simulink library "findTargetPathParameter"  (R2022a)
settings: Solver=VariableStepAuto  StartTime=0.0  StopTime=10.0  RelTol=1e-3
undefined symbols (not defined in the file or in its folder): convergeTol
libraries: calcDistanceFromPath x4, calcPathLengthOverRange x3
settings Model: Creator=Ayaz  LastModifiedBy=lhill8
settings SolverCC: AlgebraicLoopSolver=TrustRegion
settings DebuggingCC: UnconnectedInputMsg=warning  UnconnectedOutputMsg=warning  UnconnectedLineMsg=warning  SFMachineParentedDataDiag=warning

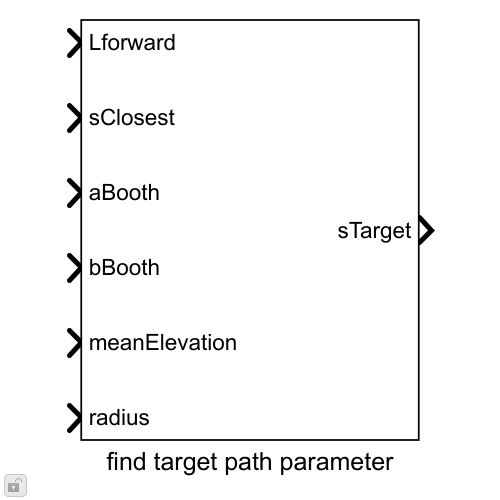
[thumbnail: Simulink's stored preview of the top-level diagram]
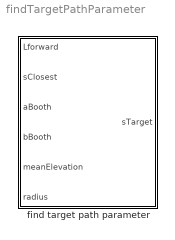
== system findTargetPathParameter ==
  find target path parameter : Subsystem  mask{maxBackward=0, maxForward=0.25, tau=0.618, convergeTol=convergeTol, MaxIters=25}
      mask prompts: maxBackward "Maximum normalized backward search"; maxForward "Maximum normalized forward search"; tau "Golden ratio"; convergeTol "Convergence tolerance"; MaxIters "Maximum number of iterations"
      mask TypeOptions maxBackward: Constant/Value
      mask TypeOptions maxForward: Constant1/Value
      mask TypeOptions tau: Golden section search/tau
      mask TypeOptions convergeTol: Golden section search/convergeTol
      mask TypeOptions MaxIters: Golden section search/MaxIters

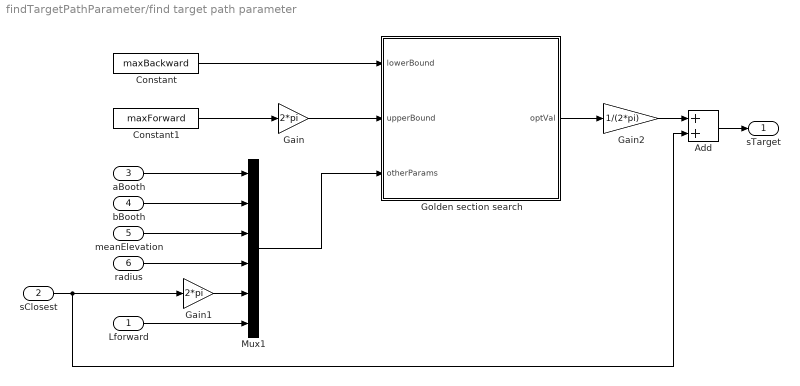
== system findTargetPathParameter/find target path parameter ==
  Lforward : Inport
  sClosest : Inport  Port=2
  aBooth : Inport  Port=3
  bBooth : Inport  Port=4
  meanElevation : Inport  Port=5
  radius : Inport  Port=6
  Add : Sum
  Constant : Constant  Value=maxBackward
  Constant1 : Constant  Value=maxForward
  Gain : Gain  Gain=2*pi
  Gain1 : Gain  Gain=2*pi
  Gain2 : Gain  Gain=1/(2*pi)
  Golden section search : Subsystem  TreatAsAtomicUnit=on  mask{tau=tau, convergeTol=convergeTol, MaxIters=25}
      mask prompts: tau "Golden ratio"; convergeTol "Convergence tolerance"; MaxIters "Maximum number of iterations"
      mask TypeOptions tau: GS initialization/tau | GS update/tau
      mask TypeOptions convergeTol: Constant/Value
      mask TypeOptions MaxIters: While Iterator/MaxIters
  Mux1 : Mux  Inputs=6
  sTarget : Outport
  wires:
  Golden section search/1(optVal) -> Gain2/1
  aBooth/1 -> Mux1/1
  radius/1 -> Mux1/4
  sClosest/1 -> Add/2, Gain1/1
  meanElevation/1 -> Mux1/3
  bBooth/1 -> Mux1/2
  Lforward/1 -> Mux1/6
  Mux1/1 -> Golden section search/3(otherParams)
  Constant/1 -> Golden section search/1(lowerBound)
  Constant1/1 -> Gain/1
  Gain/1 -> Golden section search/2(upperBound)
  Gain1/1 -> Mux1/5
  Gain2/1 -> Add/1
  Add/1 -> sTarget/1

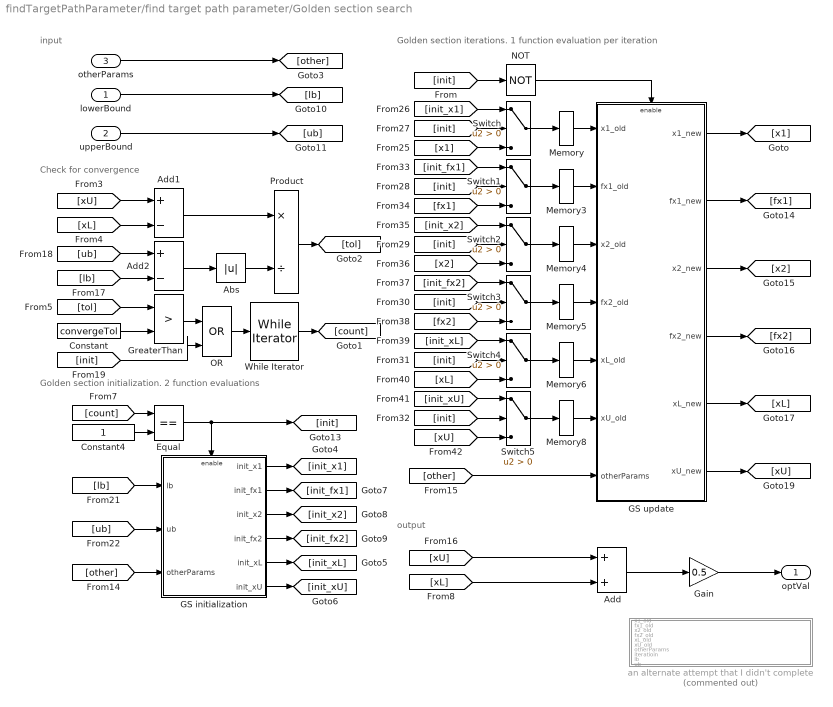
== system findTargetPathParameter/find target path parameter/Golden section search ==
  note: input
  note: output
  note: Golden section iterations. 1 function evaluation per iteration
  note: Golden section initialization. 2 function evaluations
  note: Check for convergence
  lowerBound : Inport
  upperBound : Inport  Port=2
  otherParams : Inport  Port=3
  Abs : Abs  SaturateOnIntegerOverflow=off
  Add : Sum
  Add1 : Sum  Inputs=+-
  Add2 : Sum  Inputs=+-
  Constant : Constant  Value=convergeTol
  Constant4 : Constant
  Equal : RelationalOperator  Operator===  OutDataTypeStr=boolean  RndMeth=Simplest  InputSameDT=off
  GS initialization : Subsystem  TreatAsAtomicUnit=on  mask{tau=tau}
      mask prompts: tau "Golden ratio"
      mask TypeOptions tau: Gain/Gain
  GS update : Subsystem  TreatAsAtomicUnit=on  mask{tau=tau}
      mask prompts: tau "Golden ratio"
      mask TypeOptions tau: Gain/Gain | Gain1/Gain
  Gain : Gain  Gain=0.5
  GreaterThan : RelationalOperator  Operator=>  OutDataTypeStr=boolean  RndMeth=Simplest  InputSameDT=off
  Memory{,3..6,8} (6 alike) : Memory  InheritSampleTime=on
  NOT : Logic  Operator=NOT  IconShape=distinctive  AllPortsSameDT=off  OutDataTypeStr=boolean
  OR : Logic  Operator=OR  IconShape=distinctive  AllPortsSameDT=off  OutDataTypeStr=boolean
  Product : Product  Inputs=*/
  Switch{,1..5} (6 alike) : Switch  Criteria=u2 > Threshold  SaturateOnIntegerOverflow=off  InputSameDT=off
  While Iterator : WhileIterator  MaxIters=MaxIters  WhileBlockType=do-while  ResetStates=reset  ShowIterationPort=on
  an alternate attempt that I didn't complete : Subsystem  Commented=on
  optVal : Outport
  wires:
  GreaterThan/1 -> OR/1
  Gain/1 -> optVal/1
  While Iterator/1 -> [count]
  [count] -> Equal/1
  Constant4/1 -> Equal/2
  Equal/1 -> [init], GS initialization/Enable
  [init] -> NOT/1
  Add/1 -> Gain/1
  GS initialization/1(init_x1) -> [init_x1]
  GS initialization/2(init_fx1) -> [init_fx1]
  GS initialization/3(init_x2) -> [init_x2]
  GS initialization/4(init_fx2) -> [init_fx2]
  GS update/1(x1_new) -> [x1]
  GS update/2(fx1_new) -> [fx1]
  GS update/3(x2_new) -> [x2]
  GS update/5(xL_new) -> [xL]
  GS update/6(xU_new) -> [xU]
  GS update/4(fx2_new) -> [fx2]
  otherParams/1 -> [other]
  GS initialization/5(init_xL) -> [init_xL]
  GS initialization/6(init_xU) -> [init_xU]
  [other] -> GS initialization/3(otherParams)
  [other] -> GS update/7(otherParams)
  lowerBound/1 -> [lb]
  upperBound/1 -> [ub]
  [lb] -> GS initialization/1(lb)
  [ub] -> GS initialization/2(ub)
  [init_x1] -> Switch/1
  [init] -> Switch/2
  [init] -> Switch1/2
  [fx1] -> Switch1/3
  [init_fx1] -> Switch1/1
  [init] -> Switch2/2
  [x2] -> Switch2/3
  [init_x2] -> Switch2/1
  [init] -> Switch3/2
  [fx2] -> Switch3/3
  [init_fx2] -> Switch3/1
  [init] -> Switch4/2
  [xL] -> Switch4/3
  [init_xL] -> Switch4/1
  [init] -> Switch5/2
  [xU] -> Switch5/3
  [init_xU] -> Switch5/1
  NOT/1 -> GS update/Enable
  [xL] -> Add/2
  [xU] -> Add/1
  [xU] -> Add1/1
  [xL] -> Add1/2
  Constant/1 -> GreaterThan/2
  [tol] -> GreaterThan/1
  Switch/1 -> Memory/1
  Switch3/1 -> Memory5/1
  Switch2/1 -> Memory4/1
  Switch1/1 -> Memory3/1
  Switch5/1 -> Memory8/1
  Switch4/1 -> Memory6/1
  [x1] -> Switch/3
  Memory/1 -> GS update/1(x1_old)
  Memory3/1 -> GS update/2(fx1_old)
  Memory5/1 -> GS update/4(fx2_old)
  Memory4/1 -> GS update/3(x2_old)
  Memory8/1 -> GS update/6(xU_old)
  Memory6/1 -> GS update/5(xL_old)
  [ub] -> Add2/1
  [lb] -> Add2/2
  Add2/1 -> Abs/1
  Add1/1 -> Product/1
  Abs/1 -> Product/2
  Product/1 -> [tol]
  [init] -> OR/2
  OR/1 -> While Iterator/1

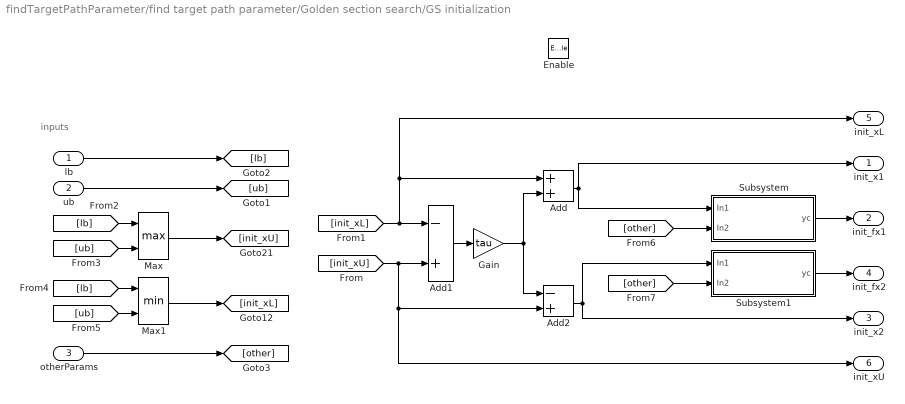
== system findTargetPathParameter/find target path parameter/Golden section search/GS initialization ==
  note: inputs
  lb : Inport
  ub : Inport  Port=2
  otherParams : Inport  Port=3
  Enable : EnablePort
  Add : Sum
  Add1 : Sum  Inputs=-+
  Add2 : Sum  Inputs=-+
  Gain : Gain  Gain=tau
  Max : MinMax  Function=max  Inputs=2
  Max1 : MinMax  Inputs=2
  Subsystem : Subsystem
  Subsystem1 : Subsystem
  init_x1 : Outport
  init_fx1 : Outport  Port=2
  init_x2 : Outport  Port=3
  init_fx2 : Outport  Port=4
  init_xL : Outport  Port=5
  init_xU : Outport  Port=6
  wires:
  Add/1 -> Subsystem/1(In1), init_x1/1
  Subsystem/1(yc) -> init_fx1/1
  Add2/1 -> init_x2/1, Subsystem1/1(In1)
  Subsystem1/1(yc) -> init_fx2/1
  Add1/1 -> Gain/1
  Gain/1 -> Add2/1, Add/2
  Max/1 -> [init_xU]
  Max1/1 -> [init_xL]
  [init_xL] -> init_xL/1, Add/1, Add1/1
  [init_xU] -> init_xU/1, Add2/2, Add1/2
  ub/1 -> [ub]
  lb/1 -> [lb]
  [lb] -> Max/1
  [ub] -> Max/2
  [lb] -> Max1/1
  [ub] -> Max1/2
  otherParams/1 -> [other]
  [other] -> Subsystem/2(In2)
  [other] -> Subsystem1/2(In2)

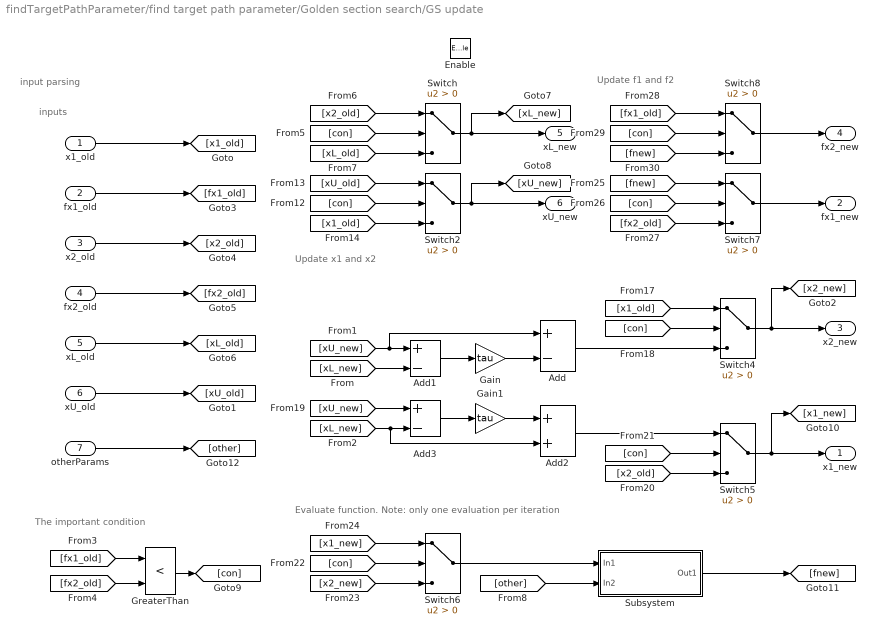
== system findTargetPathParameter/find target path parameter/Golden section search/GS update ==
  note: Evaluate function. Note: only one evaluation per iteration
  note: Update f1 and f2
  note: Update x1 and x2
  note: input parsing
  note: inputs
  note: The important condition
  x1_old : Inport
  fx1_old : Inport  Port=2
  x2_old : Inport  Port=3
  fx2_old : Inport  Port=4
  xL_old : Inport  Port=5
  xU_old : Inport  Port=6
  otherParams : Inport  Port=7
  Enable : EnablePort
  Add : Sum  Inputs=+-
  Add1 : Sum  Inputs=+-
  Add2 : Sum
  Add3 : Sum  Inputs=+-
  Gain : Gain  Gain=tau
  Gain1 : Gain  Gain=tau
  GreaterThan : RelationalOperator  Operator=<  OutDataTypeStr=boolean  RndMeth=Simplest  InputSameDT=off
  Subsystem : Subsystem
  Switch{,2,4..8} (7 alike) : Switch  Criteria=u2 > Threshold  SaturateOnIntegerOverflow=off  InputSameDT=off
  x1_new : Outport
  fx1_new : Outport  Port=2
  x2_new : Outport  Port=3
  fx2_new : Outport  Port=4
  xL_new : Outport  Port=5
  xU_new : Outport  Port=6
  wires:
  Add1/1 -> Gain/1
  Add/1 -> Switch4/3
  [xL_new] -> Add1/2
  [xU_new] -> Add/1, Add1/1
  xU_old/1 -> [xU_old]
  fx1_old/1 -> [fx1_old]
  x2_old/1 -> [x2_old]
  fx2_old/1 -> [fx2_old]
  xL_old/1 -> [xL_old]
  [fx1_old] -> GreaterThan/1
  [fx2_old] -> GreaterThan/2
  GreaterThan/1 -> [con]
  [con] -> Switch/2
  Switch/1 -> [xL_new], xL_new/1
  [x2_old] -> Switch/1
  [xL_old] -> Switch/3
  Switch4/1 -> [x2_new], x2_new/1
  [x1_old] -> Switch4/1
  [con] -> Switch4/2
  Gain/1 -> Add/2
  [con] -> Switch5/2
  Switch5/1 -> [x1_new], x1_new/1
  [xU_new] -> Add3/1
  Add3/1 -> Gain1/1
  [xL_new] -> Add2/2, Add3/2
  Add2/1 -> Switch5/1
  Gain1/1 -> Add2/1
  [x2_old] -> Switch5/3
  [con] -> Switch6/2
  [x1_new] -> Switch6/1
  [x2_new] -> Switch6/3
  Switch6/1 -> Subsystem/1(In1)
  Subsystem/1(Out1) -> [fnew]
  [fnew] -> Switch7/1
  [con] -> Switch7/2
  [fx2_old] -> Switch7/3
  Switch7/1 -> fx1_new/1
  Switch8/1 -> fx2_new/1
  [fx1_old] -> Switch8/1
  [con] -> Switch8/2
  [fnew] -> Switch8/3
  otherParams/1 -> [other]
  [x1_old] -> Switch2/3
  [xU_old] -> Switch2/1
  [con] -> Switch2/2
  Switch2/1 -> [xU_new], xU_new/1
  [other] -> Subsystem/2(In2)
  x1_old/1 -> [x1_old]

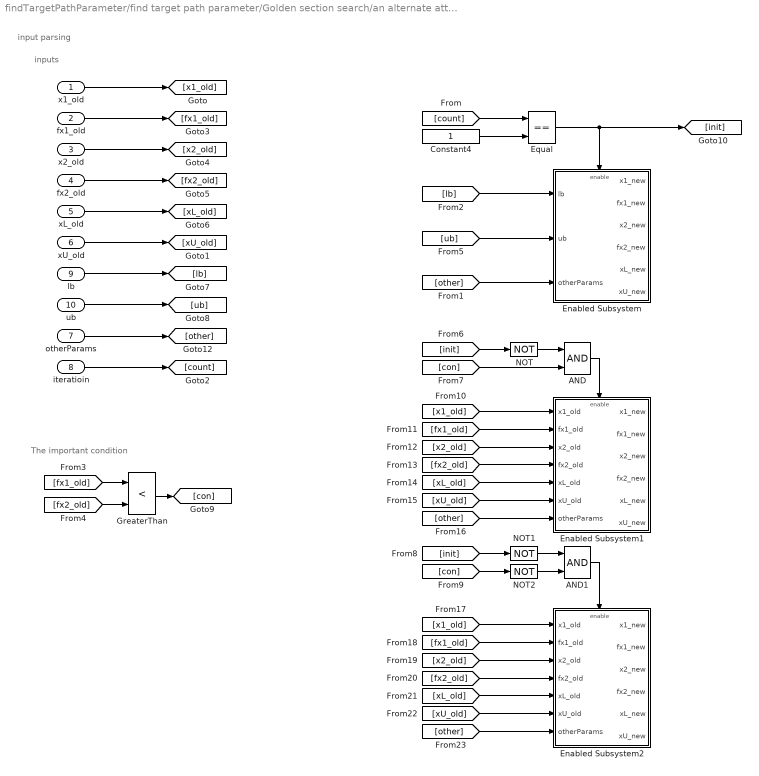
== system findTargetPathParameter/find target path parameter/Golden section search/an alternate attempt that I didn't complete ==
  note: inputs
  note: The important condition
  note: input parsing
  x1_old : Inport
  fx1_old : Inport  Port=2
  x2_old : Inport  Port=3
  fx2_old : Inport  Port=4
  xL_old : Inport  Port=5
  xU_old : Inport  Port=6
  otherParams : Inport  Port=7
  iteratioin : Inport  Port=8
  lb : Inport  Port=9
  ub : Inport  Port=10
  AND : Logic  IconShape=distinctive  AllPortsSameDT=off  OutDataTypeStr=boolean
  AND1 : Logic  IconShape=distinctive  AllPortsSameDT=off  OutDataTypeStr=boolean
  Constant4 : Constant
  Enabled Subsystem : Subsystem  TreatAsAtomicUnit=on
  Enabled Subsystem1 : Subsystem  TreatAsAtomicUnit=on
  Enabled Subsystem2 : Subsystem  TreatAsAtomicUnit=on
  Equal : RelationalOperator  Operator===  OutDataTypeStr=boolean  RndMeth=Simplest  InputSameDT=off
  GreaterThan : RelationalOperator  Operator=<  OutDataTypeStr=boolean  RndMeth=Simplest  InputSameDT=off
  NOT : Logic  Operator=NOT  IconShape=distinctive  AllPortsSameDT=off  OutDataTypeStr=boolean
  NOT1 : Logic  Operator=NOT  IconShape=distinctive  AllPortsSameDT=off  OutDataTypeStr=boolean
  NOT2 : Logic  Operator=NOT  IconShape=distinctive  AllPortsSameDT=off  OutDataTypeStr=boolean
  wires:
  x1_old/1 -> [x1_old]
  fx2_old/1 -> [fx2_old]
  x2_old/1 -> [x2_old]
  fx1_old/1 -> [fx1_old]
  otherParams/1 -> [other]
  xU_old/1 -> [xU_old]
  xL_old/1 -> [xL_old]
  iteratioin/1 -> [count]
  Constant4/1 -> Equal/2
  [count] -> Equal/1
  Equal/1 -> [init], Enabled Subsystem/Enable
  [other] -> Enabled Subsystem/3(otherParams)
  [fx2_old] -> GreaterThan/2
  [fx1_old] -> GreaterThan/1
  GreaterThan/1 -> [con]
  lb/1 -> [lb]
  ub/1 -> [ub]
  [lb] -> Enabled Subsystem/1(lb)
  [ub] -> Enabled Subsystem/2(ub)
  [init] -> NOT/1
  NOT/1 -> AND/1
  [con] -> AND/2
  AND/1 -> Enabled Subsystem1/Enable
  NOT1/1 -> AND1/1
  AND1/1 -> Enabled Subsystem2/Enable
  [con] -> NOT2/1
  [init] -> NOT1/1
  NOT2/1 -> AND1/2
  [x1_old] -> Enabled Subsystem1/1(x1_old)
  [fx1_old] -> Enabled Subsystem1/2(fx1_old)
  [x2_old] -> Enabled Subsystem1/3(x2_old)
  [fx2_old] -> Enabled Subsystem1/4(fx2_old)
  [xL_old] -> Enabled Subsystem1/5(xL_old)
  [xU_old] -> Enabled Subsystem1/6(xU_old)
  [other] -> Enabled Subsystem1/7(otherParams)
  [x2_old] -> Enabled Subsystem2/3(x2_old)
  [xU_old] -> Enabled Subsystem2/6(xU_old)
  [x1_old] -> Enabled Subsystem2/1(x1_old)
  [fx1_old] -> Enabled Subsystem2/2(fx1_old)
  [fx2_old] -> Enabled Subsystem2/4(fx2_old)
  [xL_old] -> Enabled Subsystem2/5(xL_old)
  [other] -> Enabled Subsystem2/7(otherParams)

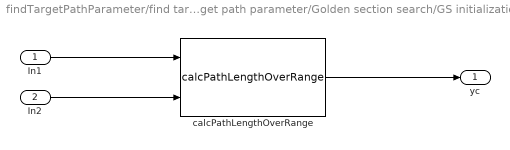
== system findTargetPathParameter/find target path parameter/Golden section search/GS initialization/Subsystem ==
  In1 : Inport
  In2 : Inport  Port=2
  calcPathLengthOverRange : calcPathLengthOverRange/calcPathLengthOverRange  SystemSampleTime=-1  VariantActivationTime=update diagram  Latency=0  AutoFrameSizeCalculation=off
  yc : Outport
  wires:
  In1/1 -> calcPathLengthOverRange/1
  In2/1 -> calcPathLengthOverRange/2
  calcPathLengthOverRange/1 -> yc/1

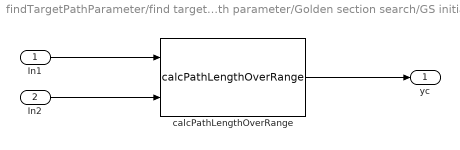
== system findTargetPathParameter/find target path parameter/Golden section search/GS initialization/Subsystem1 ==
  In1 : Inport
  In2 : Inport  Port=2
  calcPathLengthOverRange : calcPathLengthOverRange/calcPathLengthOverRange  SystemSampleTime=-1  VariantActivationTime=update diagram  Latency=0  AutoFrameSizeCalculation=off
  yc : Outport
  wires:
  In1/1 -> calcPathLengthOverRange/1
  In2/1 -> calcPathLengthOverRange/2
  calcPathLengthOverRange/1 -> yc/1

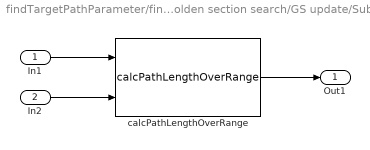
== system findTargetPathParameter/find target path parameter/Golden section search/GS update/Subsystem ==
  In1 : Inport
  In2 : Inport  Port=2
  calcPathLengthOverRange : calcPathLengthOverRange/calcPathLengthOverRange  SystemSampleTime=-1  VariantActivationTime=update diagram  Latency=0  AutoFrameSizeCalculation=off
  Out1 : Outport
  wires:
  In2/1 -> calcPathLengthOverRange/2
  In1/1 -> calcPathLengthOverRange/1
  calcPathLengthOverRange/1 -> Out1/1

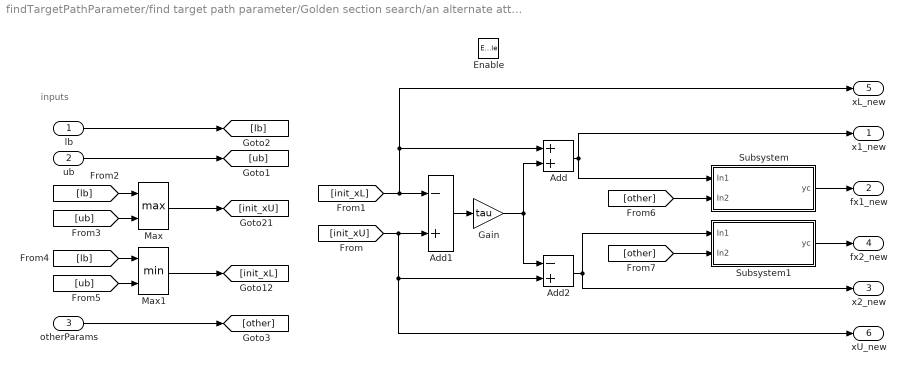
== system findTargetPathParameter/find target path parameter/Golden section search/an alternate attempt that I didn't complete/Enabled Subsystem ==
  note: inputs
  lb : Inport
  ub : Inport  Port=2
  otherParams : Inport  Port=3
  Enable : EnablePort
  Add : Sum
  Add1 : Sum  Inputs=-+
  Add2 : Sum  Inputs=-+
  Gain : Gain  Gain=tau
  Max : MinMax  Function=max  Inputs=2
  Max1 : MinMax  Inputs=2
  Subsystem : Subsystem
  Subsystem1 : Subsystem
  x1_new : Outport
  fx1_new : Outport  Port=2
  x2_new : Outport  Port=3
  fx2_new : Outport  Port=4
  xL_new : Outport  Port=5
  xU_new : Outport  Port=6
  wires:
  Max/1 -> [init_xU]
  [lb] -> Max/1
  ub/1 -> [ub]
  Max1/1 -> [init_xL]
  [ub] -> Max1/2
  Add1/1 -> Gain/1
  [ub] -> Max/2
  Add/1 -> x1_new/1, Subsystem/1(In1)
  Gain/1 -> Add2/1, Add/2
  [lb] -> Max1/1
  Add2/1 -> x2_new/1, Subsystem1/1(In1)
  [other] -> Subsystem/2(In2)
  Subsystem/1(yc) -> fx1_new/1
  [init_xL] -> xL_new/1, Add/1, Add1/1
  [init_xU] -> xU_new/1, Add2/2, Add1/2
  [other] -> Subsystem1/2(In2)
  Subsystem1/1(yc) -> fx2_new/1
  lb/1 -> [lb]
  otherParams/1 -> [other]

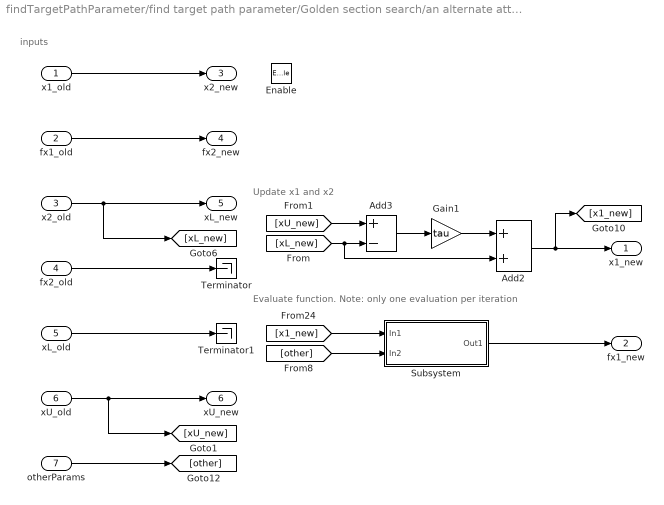
== system findTargetPathParameter/find target path parameter/Golden section search/an alternate attempt that I didn't complete/Enabled Subsystem1 ==
  note: Evaluate function. Note: only one evaluation per iteration
  note: Update x1 and x2
  note: inputs
  x1_old : Inport
  fx1_old : Inport  Port=2
  x2_old : Inport  Port=3
  fx2_old : Inport  Port=4
  xL_old : Inport  Port=5
  xU_old : Inport  Port=6
  otherParams : Inport  Port=7
  Enable : EnablePort
  Add2 : Sum
  Add3 : Sum  Inputs=+-
  Gain1 : Gain  Gain=tau
  Subsystem : Subsystem
  Terminator : Terminator
  Terminator1 : Terminator
  x1_new : Outport
  fx1_new : Outport  Port=2
  x2_new : Outport  Port=3
  fx2_new : Outport  Port=4
  xL_new : Outport  Port=5
  xU_new : Outport  Port=6
  wires:
  [other] -> Subsystem/2(In2)
  [xU_new] -> Add3/1
  Add3/1 -> Gain1/1
  Add2/1 -> x1_new/1, [x1_new]
  [xL_new] -> Add2/2, Add3/2
  [x1_new] -> Subsystem/1(In1)
  Subsystem/1(Out1) -> fx1_new/1
  Gain1/1 -> Add2/1
  x2_old/1 -> [xL_new], xL_new/1
  x1_old/1 -> x2_new/1
  fx1_old/1 -> fx2_new/1
  otherParams/1 -> [other]
  xU_old/1 -> [xU_new], xU_new/1
  fx2_old/1 -> Terminator/1
  xL_old/1 -> Terminator1/1

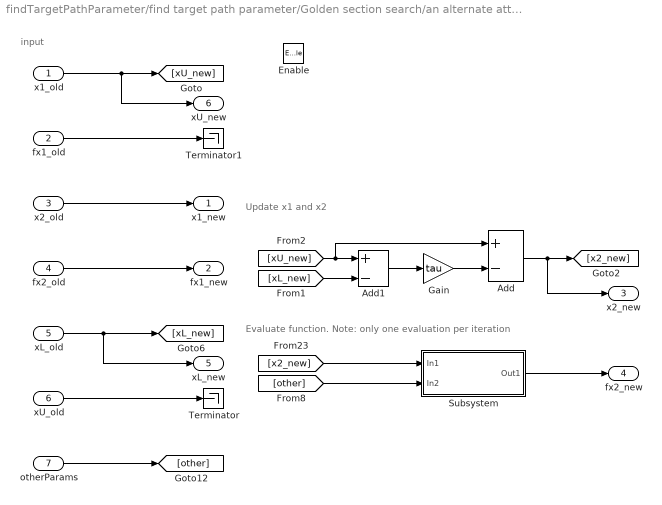
== system findTargetPathParameter/find target path parameter/Golden section search/an alternate attempt that I didn't complete/Enabled Subsystem2 ==
  note: Evaluate function. Note: only one evaluation per iteration
  note: Update x1 and x2
  note: input
  x1_old : Inport
  fx1_old : Inport  Port=2
  x2_old : Inport  Port=3
  fx2_old : Inport  Port=4
  xL_old : Inport  Port=5
  xU_old : Inport  Port=6
  otherParams : Inport  Port=7
  Enable : EnablePort
  Add : Sum  Inputs=+-
  Add1 : Sum  Inputs=+-
  Gain : Gain  Gain=tau
  Subsystem : Subsystem
  Terminator : Terminator
  Terminator1 : Terminator
  x1_new : Outport
  fx1_new : Outport  Port=2
  x2_new : Outport  Port=3
  fx2_new : Outport  Port=4
  xL_new : Outport  Port=5
  xU_new : Outport  Port=6
  wires:
  [other] -> Subsystem/2(In2)
  xU_old/1 -> Terminator/1
  Gain/1 -> Add/2
  x2_old/1 -> x1_new/1
  [x2_new] -> Subsystem/1(In1)
  fx1_old/1 -> Terminator1/1
  fx2_old/1 -> fx1_new/1
  xL_old/1 -> xL_new/1, [xL_new]
  Subsystem/1(Out1) -> fx2_new/1
  Add1/1 -> Gain/1
  otherParams/1 -> [other]
  [xU_new] -> Add/1, Add1/1
  x1_old/1 -> xU_new/1, [xU_new]
  [xL_new] -> Add1/2
  Add/1 -> x2_new/1, [x2_new]

== system findTargetPathParameter/find target path parameter/Golden section search/an alternate attempt that I didn't complete/Enabled Subsystem/Subsystem ==
  In1 : Inport
  In2 : Inport  Port=2
  calcDistanceFromPath : calcDistanceFromPath/calcDistanceFromPath  SystemSampleTime=-1  VariantActivationTime=update diagram  Latency=0  AutoFrameSizeCalculation=off
  yc : Outport
  wires:
  In1/1 -> calcDistanceFromPath/1
  In2/1 -> calcDistanceFromPath/2
  calcDistanceFromPath/1 -> yc/1

== system findTargetPathParameter/find target path parameter/Golden section search/an alternate attempt that I didn't complete/Enabled Subsystem/Subsystem1 ==
  In1 : Inport
  In2 : Inport  Port=2
  calcDistanceFromPath : calcDistanceFromPath/calcDistanceFromPath  SystemSampleTime=-1  VariantActivationTime=update diagram  Latency=0  AutoFrameSizeCalculation=off
  yc : Outport
  wires:
  In1/1 -> calcDistanceFromPath/1
  In2/1 -> calcDistanceFromPath/2
  calcDistanceFromPath/1 -> yc/1

== system findTargetPathParameter/find target path parameter/Golden section search/an alternate attempt that I didn't complete/Enabled Subsystem1/Subsystem ==
  In1 : Inport
  In2 : Inport  Port=2
  calcDistanceFromPath : calcDistanceFromPath/calcDistanceFromPath  SystemSampleTime=-1  VariantActivationTime=update diagram  Latency=0  AutoFrameSizeCalculation=off
  Out1 : Outport
  wires:
  In2/1 -> calcDistanceFromPath/2
  In1/1 -> calcDistanceFromPath/1
  calcDistanceFromPath/1 -> Out1/1

== system findTargetPathParameter/find target path parameter/Golden section search/an alternate attempt that I didn't complete/Enabled Subsystem2/Subsystem ==
  In1 : Inport
  In2 : Inport  Port=2
  calcDistanceFromPath : calcDistanceFromPath/calcDistanceFromPath  SystemSampleTime=-1  VariantActivationTime=update diagram  Latency=0  AutoFrameSizeCalculation=off
  Out1 : Outport
  wires:
  In2/1 -> calcDistanceFromPath/2
  In1/1 -> calcDistanceFromPath/1
  calcDistanceFromPath/1 -> Out1/1
